simulink model "inverted_pendulum_nonlinear"  (R2023b)
settings: Solver=VariableStepAuto  StartTime=0.0  StopTime=0.5  RelTol=1e-3
settings Model: Creator=tirio  LastModifiedBy=mamad
settings SolverCC: AlgebraicLoopSolver=TrustRegion
settings DataIOCC: ExternalInput=[0 0]  InitialState=[]  LoadInitialState=on
settings OptimizationCC: DefaultParameterBehavior=Inlined  BufferReuse=off
settings DebuggingCC: UnconnectedInputMsg=warning  UnconnectedOutputMsg=warning  UnconnectedLineMsg=warning  InitInArrayFormatMsg=none
settings ModelReferenceCC: EnableRefExpFcnMdlSchedulingChecks=on
settings RTWCC: DLArmComputeVersion=19.05

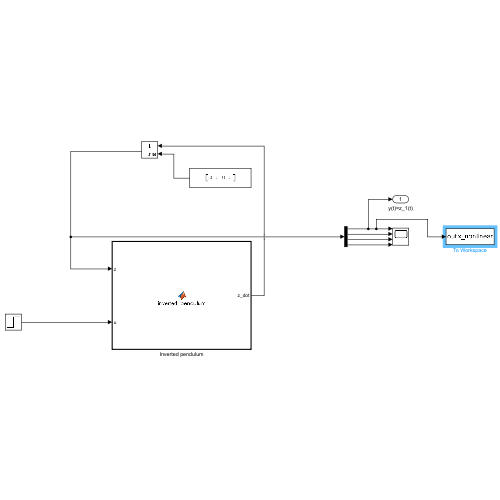
[thumbnail: Simulink's stored preview of the top-level diagram]
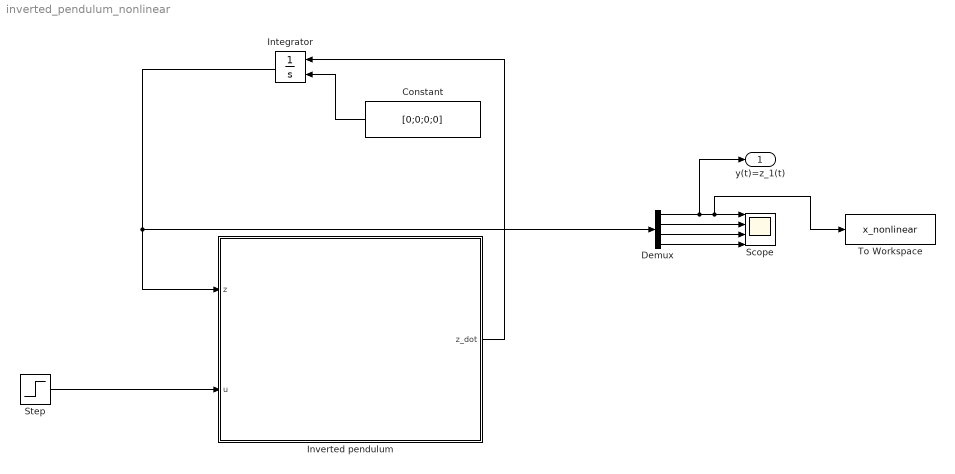
== system inverted_pendulum_nonlinear ==
  Constant : Constant  Value=[0;0;0;0]
  Demux : Demux
  Integrator : Integrator  InitialConditionSource=external
  Inverted pendulum : MATLAB Function  TreatAsAtomicUnit=on
  Scope : Scope  NumInputPorts=4
  Step : Step  SampleTime=0
  To Workspace : ToWorkspace  VariableName=x_nonlinear  SaveFormat=Timeseries  SampleTime=-1
  y(t)=z_1(t) : Outport
  wires:
  Inverted pendulum/1(z_dot) -> Integrator/1
  Integrator/1 -> Demux/1, Inverted pendulum/1(z)
  Constant/1 -> Integrator/2
  Demux/1 -> y(t)=z_1(t)/1, To Workspace/1, Scope/1
  Demux/2 -> Scope/2
  Demux/3 -> Scope/3
  Demux/4 -> Scope/4
  Step/1 -> Inverted pendulum/2(u)

== matlab function inverted_pendulum_nonlinear/Inverted pendulum ==
  data: z input; u input; z_dot output
function z_dot = inverted_pendulum(z, u)
    % Parameters
    M = 2;      % Mass of the cart [kg]
    m = 0.5;    % Mass of the pendulum [kg]
    b = 0.1;    % Friction coefficient [N·s/m]
    L = 0.3;    % Length of the pendulum [m]
    g = 9.81;   % Gravitational acceleration [m/s^2]

    % State variables
    z1 = z(1); % x (cart position)
    z2 = z(2); % x_dot (cart velocity)
    z3 = z(3); % theta (pendulum angle)
    z4 = z(4); % theta_dot (pendulum angular velocity)

    % State derivatives
    z1_dot = z2; % dx/dt = x_dot
    
    cos_z3 = cos(z3);
    sin_z3 = sin(z3);
    
    % Denominator term for the equations
    denominator = L^2 * (M + m * (1 - cos_z3^2));
    
    % Equation for the acceleration of the cart (x_double_dot)
    z2_dot = (-m^2 * L^2 * g * cos_z3 * sin_z3 + m * L^2 * (m * L * z4^2 * sin_z3 - b * z2) + m * L^2 * u) / denominator;
    
    z3_dot = z4; % dtheta/dt = theta_dot
    
    % Equation for the angular acceleration of the pendulum (theta_double_dot)
    z4_dot = ((m + M) * g * L * sin_z3 - m * L * cos_z3 * (m * L * z4^2 * sin_z3 - b * z2) + m * L * cos_z3 * u) / denominator;

    % Return state derivatives as a column vector
    z_dot = [z1_dot; z2_dot; z3_dot; z4_dot];
end
